simulink model "AdaptiveCVSG"  (R2024b)
settings: Solver=ode4  StartTime=0.0  StopTime=60  FixedStep=1e-5  RelTol=1e-3
values from neighbouring files (symbols this model uses):
  mu = [6.21887134042 12.8843826697 23.6426615734 36.1444015647 49.5413580793 62.7022204476 75.4864006017 87.7683458466 99.0601107857 109.575241947 118.563685645 126.700169925 ... (200 elements, 1x200)]    [ann_model_params.mat]
  sigma = [10.4496327183 11.1148041158 11.7472409052 11.8906256492 12.3094874175 12.8461052911 13.270989651 13.5844531441 13.6128801345 13.7374243761 13.6590800387 13.618168837 ... (200 elements, 1x200)]    [ann_model_params.mat]
undefined symbols (not defined in the file or in its folder): Filter, Ls, params
libraries: neural x14, spsCurrentMeasurementLib x6, spsParallelRLCBranchLib x6, spsIGBTDiodeLib x6, spsSeriesRLCBranchLib x6, simulink x4, spsVoltageMeasurementLib x4, spsVariableInductorLib x3, spsVariableResistorLib x3, spsMeanLib x2, spsDCVoltageSourceLib x1, spsThreePhaseSourceLib x1
(part 2 of 4)

== system AdaptiveCVSG/ANN_based GIE/Feed-Forward Neural Network/Process Input 1 ==
  x : Inport  PortDimensions=200
      mask Display: e = 0.06;c1 = [120 230 180]/255;c2 = ([120 230 180]+0)/(256+128);c3 = ([120 230 180]+128)/(256+128);patch([0 1 1 0],[0 0 1 1],c1);patch([0 1 1 1-e 1-e 0+e],[0 0 1 1-e 0+e 0+e],c2);patch([0 0 1 1-e 0+e 0+e],[0 1 1 1-e 1-e 0+e],c3);plot([0 1 1 0 0],[0 0 1 1 0]);
  mapminmax : neural/Processing Functions/mapminmax  xmin=[-1.92900329932091740836597182351;-2.14909526938133810247677502048;-3.00059736148077060846617314382;-3.88226698958890148460909585992;-4.85432914581085395155923833954;-5.52110278337038362650446288171;-6.30303679731106214489955164026;-7.04637386001331034179884227342;-7.89813916639709479028397254297;-9.0421249647800223669946717564;-9.63934294675331493351677636383;-9.93308860838287621675135596888;-10.6656556398997075518764177104;-11.0058993311379023083418360329;-11.3008961317731078111137321685;-12.1007132517375470825982120004;-11.878890270093764414127690543;-11.592769590247904432089853799;-10.241859049854243224331185047;-9.4290645304381079938593757106;-9.40930077866315528467566764448;-9.35333172927286327080764749553;-9.58262714790588887581179733388;-10.2093977541566278688378588413;-10.1367281885514284311966548557;-10.4043473998477775666060551885;-10.2392830151796481175097142113;-10.6430167171960263772234611679;-11.0280708059018088817992975237;-11.0036569909669630362714087823;-10.9425865444079075672334511182;-11.4612147810359985555805906188;-10.6203244712784456993404091918;-10.3059459141534137671669668634;-10.0926400801501952031458131387;-9.42930784664710053277758561308;-9.62527316366250040857721614884;-10.1402313188110984043532880605;-10.1263207685799887514122019638;-10.6024795142187375773801250034;-11.3215101726019309325010908651;-11.862025956411695659653560142;-12.5046365523365921035292558372;-12.7372085285390479469924684963;-12.7105900723294045207012459286;-13.0015306663624752303576315171;-12.6243763211676665036975464318;-11.8197768277611654497150084353;-11.064168318535658741552651918;-11.2392939390002748467622950557;-12.0165348296840388542250366299;-11.3109236993903987666953980806;-10.479718570447722925109701464;-9.75662721154903245235345821129;-8.65023941358128034551100427052;-8.52234760215667641602976800641;-7.15206375459950738360248578829;-5.97652735643262023046418107697;-5.18933156417944907445871649543;-4.7580792635253894573565958126;-5.2717597398462414659547903284;-4.45840365845997688154511706671;-4.17758868555159157409661929705;-4.36068697630298363066003730637;-4.41021858512980724498220297392;-3.89705057346397465423137873586;-3.79608784656931774748045427259;-4.05648042347665782614285490126;-3.39731850300812521226134776953;-3.03854050336750391991813557979;-2.74151583180257407690305626602;-2.6614005702490346472188775806;-2.67086783786861525769040781597;-2.16388646702857467829517190694;-2.23538133230434921117080193653;-2.13570261192103982850198917731;-2.16221435559382513247328461148;-1.95449735809152125298737701087;-1.9925908789232595896834254745;-1.93100795810394632034956430289;-1.96076349580406383843467210681;-1.819851391956897046497942938;-1.83621458162190243079692208994;-1.88612163161292190061146811786;-1.7662895506232163533866241778;-1.7463822495029426296042629474;-2.02216498086480678253451515047;-1.95374866319288886806759819592;-2.00570532415499513945178478025;-2.05299115102334317484178427549;-2.02587947423735537100242254382;-2.11485878248150749314504537324;-1.63073498997473520510936850769;-1.53953666584059867261657927884;-1.36172115202347887574774176755;-1.40067554248136616479314398021;-1.41982717079746478816559829284;-1.54133263573998613438220672833;-1.72843672658008129516815643001;-2.29909188345499471139987690549;-1.81163454558134517924372630659;-1.86299567753332406816468846955;-1.94993088311909223975249005889;-1.90604739745979911980100496294;-1.98496683313290955830154871364;-2.10211060723876874689608484914;-2.07046471570735191036760625138;-2.16058500306123768552879482741;-3.15813878078631082857441469969;-4.43702633219255204721775953658;-5.73585134390442163976331357844;-6.70514943066685642492075203336;-7.25898790653770920044962622342;-7.51206655462417849378198297927;-7.5330594807399657852897689736;-7.40849278443520375958541990258;-7.32057957280913651487708193599;-7.29731779910986588788546214346;-7.46484733741432293641082651448;-7.88927649453449486571798843215;-8.35924346957890840315030800411 ...(+2602 chars)]  xmax=[12.1731383470790994749677338405;11.4217849696417168559037236264;10.5866102474744749883939221036;9.76896385847462767060278565623;8.9285316084090489141544821905;8.09937654822854646852192672668;7.28770670081553539887408987852;5.76807215695953345857560634613;5.06690322989022057242891605711;5.3852806700348665458477626089;5.22039852156496220203507618862;4.3621380860029974613212289114;4.4405648185871857691608965979;4.4243559411582022988795870333;3.92042134016033338994589030335;4.00672712472972225583589533926;3.83225217628459580154753894021;4.12489922220839577704509792966;3.53071010811389829342488155817;2.87345496072105355267467530211;2.75518092538618475373368710279;2.69396657206651424232290992222;2.39629462905043233433843852254;2.51522488503340024834642463247;2.2241298063119590011638138094;2.0601687367888956714523374103;2.39490064775305411259864740714;2.02315622363368419200924108736;1.88067716234882853498788790603;1.69941134548613037580366835755;1.91052874589280174966177128226;1.60622065500114707958800863707;1.90086732439964034568902206956;1.53672732198446593265828141739;1.42803194696356583470731038688;1.83422473299455002226920896646;2.0915725854207902756343173678;2.11145545104355303323018233641;2.35388842096815542603849280567;2.14880975843305854766640550224;2.2588641197253260806121488713;1.98560602448002820885619712499;1.89416658064162146679620946088;1.71197346528230553985849837773;1.56434092444995620496683841338;1.69667226298795381644879398664;1.41156699522626660758817251917;1.61725921429473906698603968835;1.68574058048742436710654146736;2.1040762998647646320193871361;2.27124292156506113471436947293;2.1458273263320957191524485097;3.0925022933902495125835230283;4.21808914090817932418531199801;4.44682808658745454266636443208;5.58423204659220306922406962258;6.18864941051316108655555581208;7.18103714529163461577354610199;7.96315096486680040754890796961;8.55205330875746128072023566347;9.47614656485096418236935278401;10.048634270852145888852646749;10.4049025738537039842412923463;11.0450694320294537931204104098;11.9587973879397573284677491756;11.8647967004098013887869456084;11.8196230894113885057095103548;11.4866428779414739835829095682;10.4263706766664530078969619353;10.0676332551880918231290706899;9.66058669409931347615838603815;9.52531630668998374744660395663;9.9548566736238868202235607896;10.0236357860932248087237894651;9.97013650745943813547000900144;10.4981306185670089092809575959;10.7854094617438605041570554022;10.961198361554998825795337325;10.9399655796325330214813220664;11.063081527027671668861330545;11.4829094763636891940450368566;11.0421747857840166773257806199;10.9365905659054014620323869167;10.6495184985152882006786967395;10.3540052666644246670557549805;9.46479040324775766634957108181;9.29414541375688152413658826845;9.77195558963003918506728950888;10.1957658943483568947385720094;10.4533802871079686269695230294;10.9695834606978923631004363415;11.7180266687308503037456830498;12.2310539794671662150449265027;12.7919065857500608984764767229;12.616993333279451050543684687;12.7262972019447602178843226284;12.6935780126519084376468526898;11.9747160102440499684917085688;11.0907251611587902573319297517;11.2282016295912203673879048438;10.2646354726630519849095435347;10.5712192057201761485885072034;10.8905883429844703158551055822;11.0272661144580794712055649143;11.104983178140702904101999593;11.1876526547556771618019411108;11.2689598166250259936305155861;11.4081949574786722934049976175;11.4410136159857138693496381165;11.2565094401724223871497088112;10.608937832435600512326345779;9.39699752131969745505557511933;7.86593365286443635397972684586;6.46312585572923659071875590598;5.21898874770863319128011426073;4.14649743044195595587098068791;3.30367089142514380739612533944;2.72442163923018210169857411529;2.348015439433543516400959561;2.56886718658197654718833291554;2.86150954365400123080576122447;3.05340482220770992327629755891;3.21003119551392668284961473546;3.42614565234944379312764795031;3.49907935223119226364474343427 ...(+2391 chars)]  ymin=-1  ymax=1
  p : Outport  PortDimensions=200
      mask Display: e = 0.06;c1 = [120 230 180]/255;c2 = ([120 230 180]+0)/(256+128);c3 = ([120 230 180]+128)/(256+128);patch([0 1 1 0],[0 0 1 1],c1);patch([0 1 1 1-e 1-e 0+e],[0 0 1 1-e 0+e 0+e],c2);patch([0 0 1 1-e 0+e 0+e],[0 1 1 1-e 1-e 0+e],c3);plot([0 1 1 0 0],[0 0 1 1 0]);
  wires:
  x/1 -> mapminmax/1
  mapminmax/1 -> p/1

== system AdaptiveCVSG/ANN_based GIE/Feed-Forward Neural Network/Process Output 1 ==
  a : Inport  PortDimensions=2
      mask Display: e = 0.06;c1 = [120 230 180]/255;c2 = ([120 230 180]+0)/(256+128);c3 = ([120 230 180]+128)/(256+128);patch([0 1 1 0],[0 0 1 1],c1);patch([0 1 1 1-e 1-e 0+e],[0 0 1 1-e 0+e 0+e],c2);patch([0 0 1 1-e 0+e 0+e],[0 1 1 1-e 1-e 0+e],c3);plot([0 1 1 0 0],[0 0 1 1 0]);
  mapminmax_reverse : neural/Processing Functions/mapminmax_reverse  xmin=[1.54061984913000005192884600547;0.483999999999999985789145284798]  xmax=[11.554648868472000344809202943;3.62999999999999989341858963598]  ymin=-1  ymax=1
  y : Outport  PortDimensions=2
      mask Display: e = 0.06;c1 = [120 230 180]/255;c2 = ([120 230 180]+0)/(256+128);c3 = ([120 230 180]+128)/(256+128);patch([0 1 1 0],[0 0 1 1],c1);patch([0 1 1 1-e 1-e 0+e],[0 0 1 1-e 0+e 0+e],c2);patch([0 0 1 1-e 0+e 0+e],[0 1 1 1-e 1-e 0+e],c3);plot([0 1 1 0 0],[0 0 1 1 0]);
  wires:
  a/1 -> mapminmax_reverse/1
  mapminmax_reverse/1 -> y/1

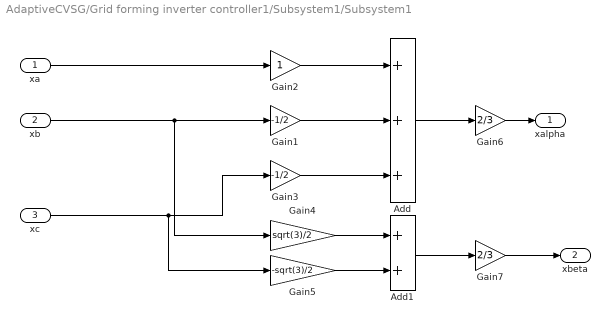
== system AdaptiveCVSG/Grid forming inverter controller1/Subsystem1/Subsystem1 ==
  xa : Inport
  xb : Inport  Port=2
  xc : Inport  Port=3
  Add : Sum  Inputs=+++
  Add1 : Sum
  Gain1 : Gain  Gain=-1/2
  Gain2 : Gain
  Gain3 : Gain  Gain=-1/2
  Gain4 : Gain  Gain=sqrt(3)/2
  Gain5 : Gain  Gain=-sqrt(3)/2
  Gain6 : Gain  Gain=2/3
  Gain7 : Gain  Gain=2/3
  xalpha : Outport  VectorParamsAs1DForOutWhenUnconnected=off
  xbeta : Outport  Port=2  VectorParamsAs1DForOutWhenUnconnected=off
  wires:
  xc/1 -> Gain5/1, Gain3/1
  Gain6/1 -> xalpha/1
  Add1/1 -> Gain7/1
  Gain3/1 -> Add/3
  Gain1/1 -> Add/2
  xb/1 -> Gain4/1, Gain1/1
  Gain5/1 -> Add1/2
  Gain2/1 -> Add/1
  Add/1 -> Gain6/1
  Gain4/1 -> Add1/1
  Gain7/1 -> xbeta/1
  xa/1 -> Gain2/1

== system AdaptiveCVSG/Grid forming inverter controller1/Subsystem1/Subsystem2 ==
  xalpha : Inport
  xbeta : Inport  Port=2
  wt : Inport  Port=3
  Fcn : Fcn  Expr=cos(u(3))*u(1)+u(2)*sin(u(3))
  Fcn1 : Fcn  Expr=-sin(u(3))*u(1)+u(2)*cos(u(3))
  Mux : Mux  Inputs=3
  xd : Outport  VectorParamsAs1DForOutWhenUnconnected=off
  xq : Outport  Port=2  VectorParamsAs1DForOutWhenUnconnected=off
  wires:
  Mux/1 -> Fcn/1, Fcn1/1
  Fcn/1 -> xd/1
  xbeta/1 -> Mux/2
  Fcn1/1 -> xq/1
  xalpha/1 -> Mux/1
  wt/1 -> Mux/3

== system AdaptiveCVSG/Grid forming inverter controller1/Subsystem3/Subsystem1 ==
  xa : Inport
  xb : Inport  Port=2
  xc : Inport  Port=3
  Add : Sum  Inputs=+++
  Add1 : Sum
  Gain1 : Gain  Gain=-1/2
  Gain2 : Gain
  Gain3 : Gain  Gain=-1/2
  Gain4 : Gain  Gain=sqrt(3)/2
  Gain5 : Gain  Gain=-sqrt(3)/2
  Gain6 : Gain  Gain=2/3
  Gain7 : Gain  Gain=2/3
  xalpha : Outport  VectorParamsAs1DForOutWhenUnconnected=off
  xbeta : Outport  Port=2  VectorParamsAs1DForOutWhenUnconnected=off
  wires:
  xa/1 -> Gain2/1
  Gain7/1 -> xbeta/1
  Gain4/1 -> Add1/1
  Add/1 -> Gain6/1
  Gain2/1 -> Add/1
  Gain5/1 -> Add1/2
  xb/1 -> Gain1/1, Gain4/1
  Gain1/1 -> Add/2
  Gain3/1 -> Add/3
  Add1/1 -> Gain7/1
  Gain6/1 -> xalpha/1
  xc/1 -> Gain3/1, Gain5/1

== system AdaptiveCVSG/Grid forming inverter controller1/Subsystem3/Subsystem2 ==
  xalpha : Inport
  xbeta : Inport  Port=2
  wt : Inport  Port=3
  Fcn : Fcn  Expr=cos(u(3))*u(1)+u(2)*sin(u(3))
  Fcn1 : Fcn  Expr=-sin(u(3))*u(1)+u(2)*cos(u(3))
  Mux : Mux  Inputs=3
  xd : Outport  VectorParamsAs1DForOutWhenUnconnected=off
  xq : Outport  Port=2  VectorParamsAs1DForOutWhenUnconnected=off
  wires:
  xalpha/1 -> Mux/1
  Fcn1/1 -> xq/1
  xbeta/1 -> Mux/2
  Fcn/1 -> xd/1
  Mux/1 -> Fcn1/1, Fcn/1
  wt/1 -> Mux/3

== system AdaptiveCVSG/Grid forming inverter controller1/Subsystem4/Subsystem1 ==
  xa : Inport
  xb : Inport  Port=2
  xc : Inport  Port=3
  Add : Sum  Inputs=+++
  Add1 : Sum
  Gain1 : Gain  Gain=-1/2
  Gain2 : Gain
  Gain3 : Gain  Gain=-1/2
  Gain4 : Gain  Gain=sqrt(3)/2
  Gain5 : Gain  Gain=-sqrt(3)/2
  Gain6 : Gain  Gain=2/3
  Gain7 : Gain  Gain=2/3
  xalpha : Outport  VectorParamsAs1DForOutWhenUnconnected=off
  xbeta : Outport  Port=2  VectorParamsAs1DForOutWhenUnconnected=off
  wires:
  xa/1 -> Gain2/1
  Gain7/1 -> xbeta/1
  Gain4/1 -> Add1/1
  Add/1 -> Gain6/1
  Gain2/1 -> Add/1
  Gain5/1 -> Add1/2
  xb/1 -> Gain1/1, Gain4/1
  Gain1/1 -> Add/2
  Gain3/1 -> Add/3
  Add1/1 -> Gain7/1
  Gain6/1 -> xalpha/1
  xc/1 -> Gain3/1, Gain5/1

== system AdaptiveCVSG/Grid forming inverter controller1/Subsystem4/Subsystem2 ==
  xalpha : Inport
  xbeta : Inport  Port=2
  wt : Inport  Port=3
  Fcn : Fcn  Expr=cos(u(3))*u(1)+u(2)*sin(u(3))
  Fcn1 : Fcn  Expr=-sin(u(3))*u(1)+u(2)*cos(u(3))
  Mux : Mux  Inputs=3
  xd : Outport  VectorParamsAs1DForOutWhenUnconnected=off
  xq : Outport  Port=2  VectorParamsAs1DForOutWhenUnconnected=off
  wires:
  wt/1 -> Mux/3
  xalpha/1 -> Mux/1
  Fcn1/1 -> xq/1
  xbeta/1 -> Mux/2
  Fcn/1 -> xd/1
  Mux/1 -> Fcn1/1, Fcn/1

== system AdaptiveCVSG/Grid forming inverter controller1/dq-abc/Subsystem2 ==
  xdq : Inport
  wt : Inport  Port=2
  Demux : Demux  Outputs=2
  Fcn2 : Fcn  Expr=u(1)*cos(u(3))-u(2)*sin(u(3))
  Fcn3 : Fcn  Expr=u(1)*sin(u(3))+u(2)*cos(u(3))
  Mux : Mux  Inputs=2
  Mux2 : Mux  Inputs=3
  xalbe : Outport  VectorParamsAs1DForOutWhenUnconnected=off
  wires:
  Mux/1 -> xalbe/1
  Fcn3/1 -> Mux/2
  Fcn2/1 -> Mux/1
  Demux/2 -> Mux2/2
  Demux/1 -> Mux2/1
  xdq/1 -> Demux/1
  wt/1 -> Mux2/3
  Mux2/1 -> Fcn3/1, Fcn2/1

== system AdaptiveCVSG/Grid forming inverter controller1/dq-abc/Subsystem3 ==
  xalbe : Inport
  Add : Sum
  Add1 : Sum
  Demux : Demux  Outputs=2
  Gain : Gain
  Gain1 : Gain  Gain=-1/2
  Gain2 : Gain  Gain=sqrt(3)/2
  Gain3 : Gain  Gain=-1/2
  Gain4 : Gain  Gain=-sqrt(3)/2
  Mux : Mux  Inputs=3
  xabc : Outport  VectorParamsAs1DForOutWhenUnconnected=off
  wires:
  xalbe/1 -> Demux/1
  Mux/1 -> xabc/1
  Gain2/1 -> Add/2
  Gain/1 -> Mux/1
  Gain4/1 -> Add1/2
  Gain3/1 -> Add1/1
  Demux/2 -> Gain4/1, Gain2/1
  Add/1 -> Mux/2
  Gain1/1 -> Add/1
  Demux/1 -> Gain3/1, Gain1/1, Gain/1
  Add1/1 -> Mux/3

== system AdaptiveCVSG/ANN_based GIE/Feed-Forward Neural Network/Layer 1/Delays 1 ==
  "p{1}" : Inport  PortDimensions=200
      mask Display: e = 0.06;c1 = [120 230 180]/255;c2 = ([120 230 180]+0)/(256+128);c3 = ([120 230 180]+128)/(256+128);patch([0 1 1 0],[0 0 1 1],c1);patch([0 1 1 1-e 1-e 0+e],[0 0 1 1-e 0+e 0+e],c2);patch([0 0 1 1-e 0+e 0+e],[0 1 1 1-e 1-e 0+e],c3);plot([0 1 1 0 0],[0 0 1 1 0]);
  mux : Mux  Inputs=1
      mask Display: e = 0.06;c1 = [120 150 230]/255;c2 = ([120 150 230]+0)/383;c3 = ([120 150 230]+128)/383;patch([0 1 1 0],[0 0 1 1],c1);patch([0 1 1 1-e 1-e 0+e],[0 0 1 1-e 0+e 0+e],c2);patch([0 0 1 1-e 0+e 0+e],[0 1 1 1-e 1-e 0+e],c3);plot([0 1 1 0 0],[0 0 1 1 0]);disp('Mux')
  "pd{1,1}" : Outport
      mask Display: e = 0.06;c1 = [120 230 180]/255;c2 = ([120 230 180]+0)/(256+128);c3 = ([120 230 180]+128)/(256+128);patch([0 1 1 0],[0 0 1 1],c1);patch([0 1 1 1-e 1-e 0+e],[0 0 1 1-e 0+e 0+e],c2);patch([0 0 1 1-e 0+e 0+e],[0 1 1 1-e 1-e 0+e],c3);plot([0 1 1 0 0],[0 0 1 1 0]);
  wires:
  "p{1}"/1 -> mux/1
  mux/1 -> "pd{1,1}"/1
